simulink model "DC_motor_spped_control_using_shount_resistence"  (R2024a)
settings: Solver=VariableStepAuto  StartTime=0.0  StopTime=10.0  RelTol=1e-3
libraries: spsIdealSwitchLib x6, spsSeriesRLCBranchLib x6, spsDCVoltageSourceLib x4, spsDCMachineLib x2, sps_lib x1
settings Model: Creator=VICTUS  LastModifiedBy=VICTUS

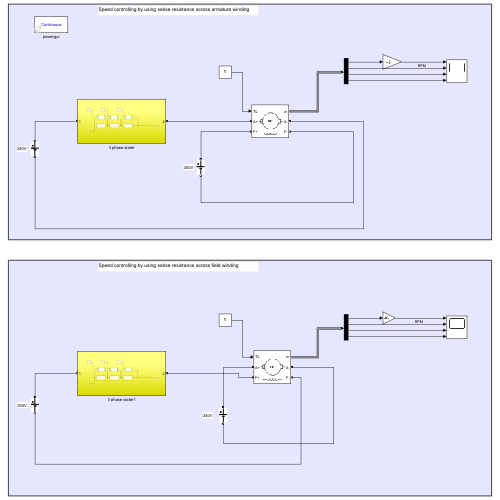
[thumbnail: Simulink's stored preview of the top-level diagram]
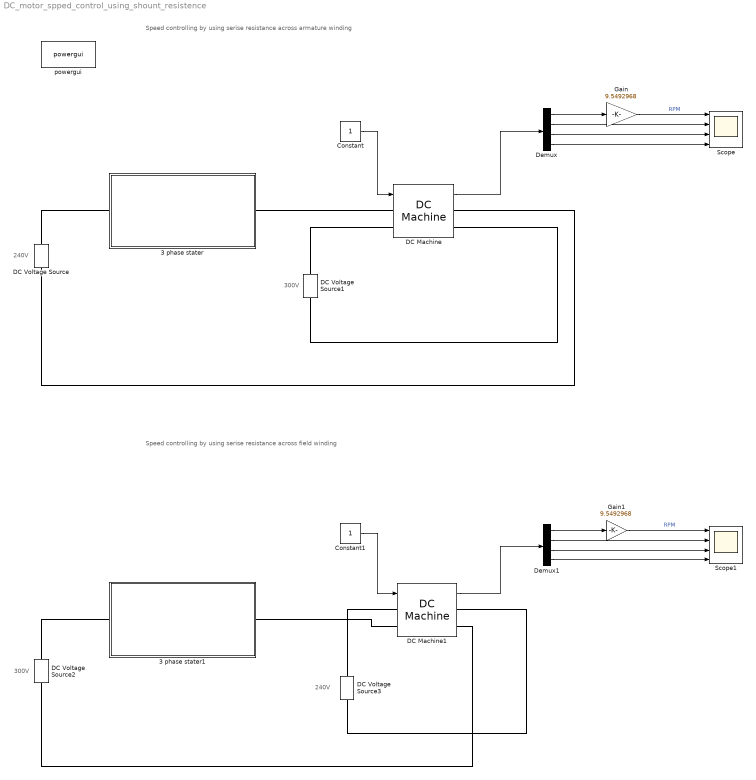
== system DC_motor_spped_control_using_shount_resistence ==
  note: Speed controlling by using serise resistance across armature winding
  note: 300V
  note: 240V
  note: Speed controlling by using serise resistance across field winding
  note: 240V
  note: 300V
  3 phase stater : Subsystem
  3 phase stater1 : Subsystem
  Constant : Constant
  Constant1 : Constant
  DC Machine : spsDCMachineLib/DC Machine  PresetModel=01: 5HP 240V 1750RPM Field:300V  MechanicalLoad=Torque TL  FieldType=Wound  ShowDetailedParameters=on  MeasurementBus=off  RLa=[2.581 0.028]  RLf=[281.2 156]  Laf=0.9483  MachineConstant=Torque constant (N.m/A)  Ke=1.8  Kt=1.8  J=0.02215  Bm=0.002953  Tf=0.5161  w0=1  Ifinit=1.06685633001422  TsPowergui=0  TsBlock=-1
  DC Machine1 : spsDCMachineLib/DC Machine  PresetModel=01: 5HP 240V 1750RPM Field:300V  MechanicalLoad=Torque TL  FieldType=Wound  ShowDetailedParameters=on  MeasurementBus=off  RLa=[2.581 0.028]  RLf=[281.2 156]  Laf=0.9483  MachineConstant=Torque constant (N.m/A)  Ke=1.8  Kt=1.8  J=0.02215  Bm=0.002953  Tf=0.5161  w0=1  Ifinit=0.842267794985998  TsPowergui=0  TsBlock=-1
  DC Voltage Source : spsDCVoltageSourceLib/DC Voltage Source  Amplitude=240  Measurements=None
  DC Voltage Source1 : spsDCVoltageSourceLib/DC Voltage Source  Amplitude=300  Measurements=None
  DC Voltage Source2 : spsDCVoltageSourceLib/DC Voltage Source  Amplitude=300  Measurements=None
  DC Voltage Source3 : spsDCVoltageSourceLib/DC Voltage Source  Amplitude=240  Measurements=None
  Demux : Demux
  Demux1 : Demux
  Gain : Gain  Gain=9.5492968
  Gain1 : Gain  Gain=9.5492968
  Scope : Scope  NumInputPorts=4
  Scope1 : Scope  NumInputPorts=4
  powergui : sps_lib/powergui  Priority=1  SimulationMode=Continuous  SampleTime=50e-6  frequency=60  Iterations=50  frequencyindice=0  Pbase=100e6  ErrMax=1e-4  UnitsV=kV  UnitsW=MW  buscounter=0  FunctionMessages=off  echomessages=off  EnableUseOfTLC=off  CurrentSourceSwitches=off  DisableSnubberDevices=off  DisableRonSwitches=off  DisableVfSwitches=off  DisplayEquations=off  AutomaticDiscreteSolvers=off  SolverType=Tustin/Backward Euler (TBE)  Interpol=off  ExternalGateDelay=off  methode=off  Ts=100  x0status=blocks  SPID=on  SwTol=0  HookPort=off  NonlinearTolerance=1e-4  nMaxIteration=100  ContinueOnMaxIteration=off  RestoreLinks=warning  ResistiveCurrentMeasurement=off  Frange=[0:2:500]  Ylog=off  Xlog=on  ShowGrid=off  save=off  variable=ZData  structure=0  ZoomFFT=off  StartTime=0.0  cycles=1  DisplayStyle=1  fundamental=60  FreqAxis=off  MaxFrequency=1000  frequencyindicesteady=1  RmsSteady=1  display=off
  wires:
  Constant/1 -> DC Machine/1
  DC Machine/1 -> Demux/1
  Demux/1 -> Gain/1
  Demux/2 -> Scope/2
  Demux/3 -> Scope/3
  Demux/4 -> Scope/4
  Gain/1 -> Scope/1  "RPM"
  Constant1/1 -> DC Machine1/1
  Demux1/1 -> Gain1/1
  Demux1/3 -> Scope1/3
  Demux1/4 -> Scope1/4
  DC Machine1/1 -> Demux1/1
  Demux1/2 -> Scope1/2
  Gain1/1 -> Scope1/1  "RPM"
  connections:
  DC Machine/RConn1 -- DC Voltage Source/LConn1
  DC Voltage Source1/RConn1 -- DC Machine/LConn2
  DC Voltage Source1/LConn1 -- DC Machine/RConn2
  DC Voltage Source2/LConn1 -- DC Machine1/RConn2
  DC Voltage Source3/RConn1 -- DC Machine1/LConn1
  DC Machine1/RConn1 -- DC Voltage Source3/LConn1
  3 phase stater/RConn1 -- DC Machine/LConn1
  DC Voltage Source/RConn1 -- 3 phase stater/LConn1
  3 phase stater1/RConn1 -- DC Machine1/LConn2
  3 phase stater1/LConn1 -- DC Voltage Source2/RConn1

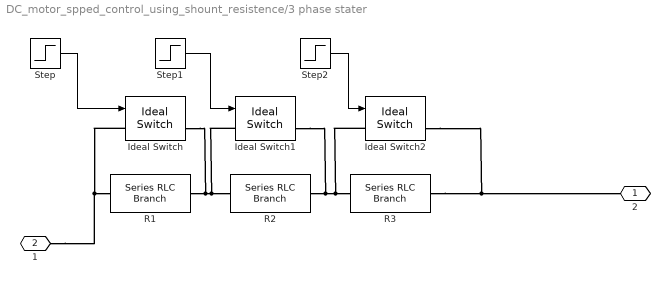
== system DC_motor_spped_control_using_shount_resistence/3 phase stater ==
  Ideal Switch : spsIdealSwitchLib/Ideal Switch  Ron=0.001  Lon=0  IC=0  Rs=1e5  Cs=inf  Measurements=on
  Ideal Switch1 : spsIdealSwitchLib/Ideal Switch  Ron=0.001  Lon=0  IC=0  Rs=1e5  Cs=inf  Measurements=on
  Ideal Switch2 : spsIdealSwitchLib/Ideal Switch  Ron=0.001  Lon=0  IC=0  Rs=1e5  Cs=inf  Measurements=on
  R1 : spsSeriesRLCBranchLib/Series RLC Branch  LConnTagsString=__new0  RConnTagsString=__new0  BranchType=R  Resistance=25  Inductance=1e-3  SetiL0=off  InitialCurrent=0  Capacitance=1e-6  Setx0=off  InitialVoltage=0  Measurements=None
  R2 : spsSeriesRLCBranchLib/Series RLC Branch  LConnTagsString=__new0  RConnTagsString=__new0  BranchType=R  Resistance=25  Inductance=1e-3  SetiL0=off  InitialCurrent=0  Capacitance=1e-6  Setx0=off  InitialVoltage=0  Measurements=None
  R3 : spsSeriesRLCBranchLib/Series RLC Branch  LConnTagsString=__new0  RConnTagsString=__new0  BranchType=R  Resistance=25  Inductance=1e-3  SetiL0=off  InitialCurrent=0  Capacitance=1e-6  Setx0=off  InitialVoltage=0  Measurements=None
  Step : Step  Time=2.5  SampleTime=0
  Step1 : Step  Time=5  SampleTime=0
  Step2 : Step  Time=7.5  SampleTime=0
  2 : PMIOPort  Side=Right
  1 : PMIOPort  Port=2  Side=Left
  wires:
  Step1/1 -> Ideal Switch1/1
  Step2/1 -> Ideal Switch2/1
  Step/1 -> Ideal Switch/1
  connections:
  Ideal Switch/LConn1 -- 1/RConn1 -- R1/LConn1
  R2/RConn1 -- Ideal Switch1/RConn1 -- Ideal Switch2/LConn1 -- R3/LConn1
  R1/RConn1 -- Ideal Switch/RConn1 -- Ideal Switch1/LConn1 -- R2/LConn1
  R3/RConn1 -- 2/RConn1 -- Ideal Switch2/RConn1

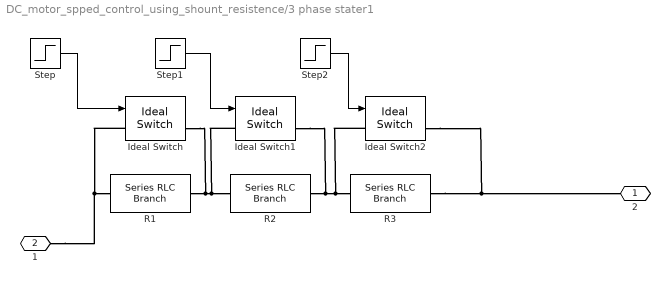
== system DC_motor_spped_control_using_shount_resistence/3 phase stater1 ==
  Ideal Switch : spsIdealSwitchLib/Ideal Switch  Ron=0.001  Lon=0  IC=0  Rs=1e5  Cs=inf  Measurements=on
  Ideal Switch1 : spsIdealSwitchLib/Ideal Switch  Ron=0.001  Lon=0  IC=0  Rs=1e5  Cs=inf  Measurements=on
  Ideal Switch2 : spsIdealSwitchLib/Ideal Switch  Ron=0.001  Lon=0  IC=0  Rs=1e5  Cs=inf  Measurements=on
  R1 : spsSeriesRLCBranchLib/Series RLC Branch  LConnTagsString=__new0  RConnTagsString=__new0  BranchType=R  Resistance=25  Inductance=1e-3  SetiL0=off  InitialCurrent=0  Capacitance=1e-6  Setx0=off  InitialVoltage=0  Measurements=None
  R2 : spsSeriesRLCBranchLib/Series RLC Branch  LConnTagsString=__new0  RConnTagsString=__new0  BranchType=R  Resistance=25  Inductance=1e-3  SetiL0=off  InitialCurrent=0  Capacitance=1e-6  Setx0=off  InitialVoltage=0  Measurements=None
  R3 : spsSeriesRLCBranchLib/Series RLC Branch  LConnTagsString=__new0  RConnTagsString=__new0  BranchType=R  Resistance=25  Inductance=1e-3  SetiL0=off  InitialCurrent=0  Capacitance=1e-6  Setx0=off  InitialVoltage=0  Measurements=None
  Step : Step  Time=2.5  SampleTime=0
  Step1 : Step  Time=5  SampleTime=0
  Step2 : Step  Time=7.5  SampleTime=0
  2 : PMIOPort  Side=Right
  1 : PMIOPort  Port=2  Side=Left
  wires:
  Step1/1 -> Ideal Switch1/1
  Step2/1 -> Ideal Switch2/1
  Step/1 -> Ideal Switch/1
  connections:
  Ideal Switch/LConn1 -- R1/LConn1 -- 1/RConn1
  R2/RConn1 -- Ideal Switch1/RConn1 -- Ideal Switch2/LConn1 -- R3/LConn1
  R1/RConn1 -- Ideal Switch/RConn1 -- Ideal Switch1/LConn1 -- R2/LConn1
  R3/RConn1 -- Ideal Switch2/RConn1 -- 2/RConn1
